simulink model "InputCond"  (R2021a)
settings: Solver=VariableStepAuto  StartTime=0.0  StopTime=inf  RelTol=1e-3
undefined symbols (not defined in the file or in its folder): aircraft, plotprob
libraries: simulink x6
settings Model: Creator=DELL  LastModifiedBy=DELL

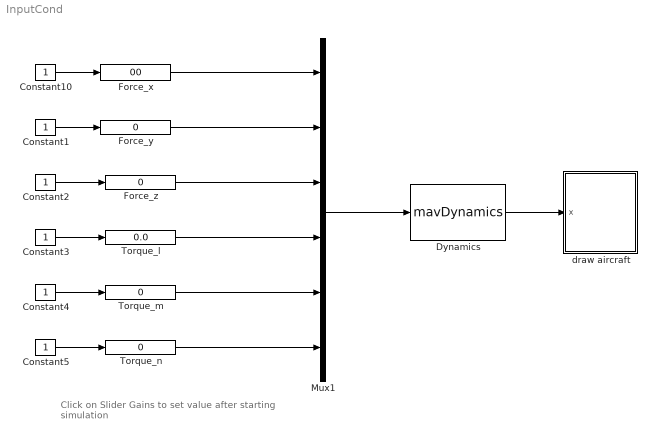
== system InputCond ==
  note: Click on Slider Gains to set value
      | after starting simulation
  Constant{1..5,10} (6 alike) : Constant
  Dynamics : S-Function  FunctionName=mavDynamics  Parameters=MAV  SFunctionDeploymentMode=off  EnableBusSupport=off
  Force_x : simulink/Math Operations/Slider Gain  gain=00  low=-1  high=10
  Force_y : simulink/Math Operations/Slider Gain  gain=0  low=-1  high=10
  Force_z : simulink/Math Operations/Slider Gain  gain=0  low=-10  high=10
  Mux1 : Mux  Inputs=6
  Torque_l : simulink/Math Operations/Slider Gain  gain=0.0  low=-10  high=10
  Torque_m : simulink/Math Operations/Slider Gain  gain=0  low=-10  high=10
  "Torque_n " : simulink/Math Operations/Slider Gain  gain=0  low=-10  high=10
  draw aircraft : Subsystem
  wires:
  Mux1/1 -> Dynamics/1
  Constant4/1 -> Torque_m/1
  Torque_m/1 -> Mux1/5
  Constant3/1 -> Torque_l/1
  Constant5/1 -> "Torque_n "/1
  Force_y/1 -> Mux1/2
  Constant2/1 -> Force_z/1
  Force_z/1 -> Mux1/3
  "Torque_n "/1 -> Mux1/6
  Torque_l/1 -> Mux1/4
  Dynamics/1 -> draw aircraft/1(x)
  Force_x/1 -> Mux1/1
  Constant1/1 -> Force_y/1
  Constant10/1 -> Force_x/1

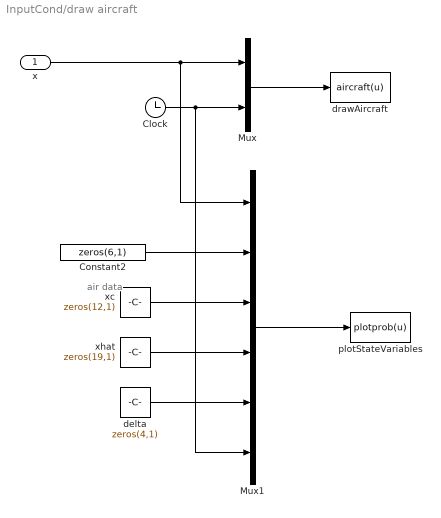
== system InputCond/draw aircraft ==
  note: air data
  x : Inport
  Clock : Clock
  Constant2 : Constant  Value=zeros(6,1)
  Mux : Mux  Inputs=2
  Mux1 : Mux  Inputs=6
  delta : Constant  Value=zeros(4,1)
  drawAircraft : MATLABFcn  MATLABFcn=aircraft(u)  OutputDimensions=0  SampleTime=0.1
  plotStateVariables : MATLABFcn  MATLABFcn=plotprob(u)  OutputDimensions=0  SampleTime=0.1
  xc : Constant  Value=zeros(12,1)
  xhat : Constant  Value=zeros(19,1)
  wires:
  Mux/1 -> drawAircraft/1
  x/1 -> Mux/1, Mux1/1
  Clock/1 -> Mux/2, Mux1/6
  Mux1/1 -> plotStateVariables/1
  xhat/1 -> Mux1/4
  xc/1 -> Mux1/3
  delta/1 -> Mux1/5
  Constant2/1 -> Mux1/2
